simulink model "reglage_PD_discret"  (Simulink 7.5)
settings: Solver=ode1  StartTime=0.0  StopTime=10.0  FixedStep=0.02  RelTol=1e-3
undefined symbols (not defined in the file): DiscIntNeverNeededParam
libraries: simulink_need_slupdate x1
settings Model: Creator=fclaveau  LastModifiedBy=fclaveau
settings OptimizationCC: InitFltsAndDblsToZero=on
settings DebuggingCC: StrictBusMsg=Warning

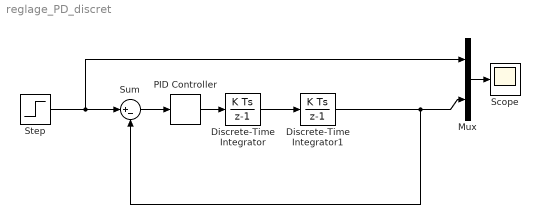
== system reglage_PD_discret ==
  Discrete-Time Integrator : DiscreteIntegrator  SampleTime=0.02  OutDataType=sfix(16)  OutScaling=2^0  ICPrevOutput=DiscIntNeverNeededParam  ICPrevScaledInput=DiscIntNeverNeededParam
  Discrete-Time Integrator1 : DiscreteIntegrator  SampleTime=0.02  OutDataType=sfix(16)  OutScaling=2^0  ICPrevOutput=DiscIntNeverNeededParam  ICPrevScaledInput=DiscIntNeverNeededParam
  Mux : Mux  Inputs=2
  PID Controller : simulink_need_slupdate/PID Controller  SystemSampleTime=-1  P=5  I=0  D=2
  Scope : Scope
  Step : Step  SampleTime=0
  Sum : Sum  Inputs=|+-  OutDataType=sfix(16)  OutScaling=2^0
  wires:
  Discrete-Time Integrator/1 -> Discrete-Time Integrator1/1
  Discrete-Time Integrator1/1 -> Sum/2, Mux/2
  Mux/1 -> Scope/1
  Step/1 -> Sum/1, Mux/1
  PID Controller/1 -> Discrete-Time Integrator/1
  Sum/1 -> PID Controller/1
